simulink model "Simulazione_OSSERVATORE"  (R2022b)
settings: Solver=VariableStepAuto  StartTime=0.0  StopTime=20  RelTol=1e-10  AbsTol=1e-10
values from neighbouring files (symbols this model uses):
  A = [ 0    0     1     0 ... (first row only)    [Tirocinio3_main.m]
  A_d = A'    [ProgettoOsservatore.m]    (also in ProgettoOsservatoreOTTIMO.m; Tirocinio3_main.m = [ 0    0     1     0)
  B = [0 0 1/m1 0 ]'    [Tirocinio3_main.m]
  B_d = C'    [ProgettoOsservatoreOTTIMO.m]    (also in Tirocinio3_main.m = [0 0 1/m1_d 0 ]')
  C = [1 0 0 0]    [Tirocinio3_main.m]
  C_d = B'    [ProgettoOsservatore.m]    (also in Tirocinio3_main.m = [1 0 0 0])
  D = 0    [Tirocinio3_main.m]
  D_d = 0    [Tirocinio3_main.m]
  M = [0 0 0 1/m2]'    [Tirocinio3_main.m]
  V_ott = K'    [Tirocinio3_main.m]
  x0 = [x1; x2; v1 ; v2 ]    [Tirocinio3_main.m]
undefined symbols (not defined in the file or in its folder): V_fast, V_slow
libraries: simulink x2
settings Model: Creator=Danilo  LastModifiedBy=Danilo

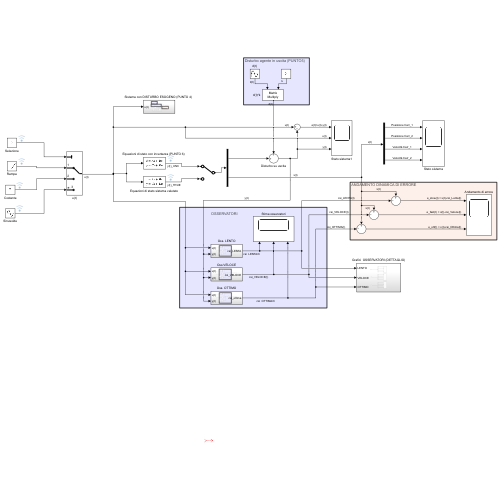
[thumbnail: Simulink's stored preview of the top-level diagram]
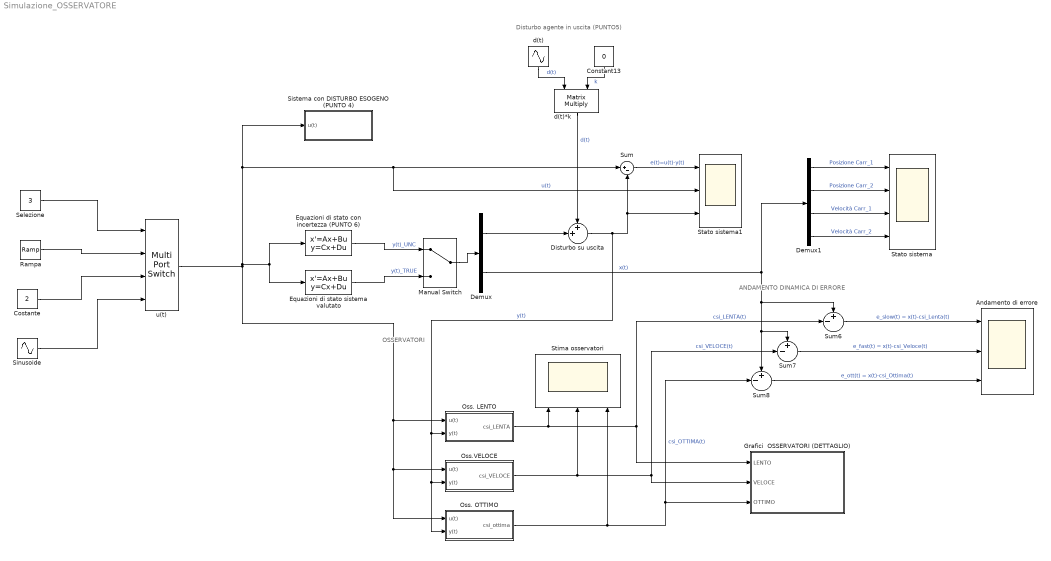
== system Simulazione_OSSERVATORE ==
  note: OSSERVATORI
  note: ANDAMENTO DINAMICA DI ERRORE
  note: Disturbo agente in uscita (PUNTO5)
  Andamento di errore : Scope  NumInputPorts=3
  Constant13 : Constant  Value=0  VectorParams1D=off
  Costante : Constant  Value=2
  Demux : Demux  Outputs=[1,4]
  Demux1 : Demux
  Disturbo su uscita : Sum  Inputs=++|
  "Equazioni di stato con incertezza (PUNTO 6)  " : StateSpace  A=A_d  B=B_d  C=[C_d ; eye(4)]  D=[D_d;zeros(4,1)]  InitialCondition=x0
  "Equazioni di stato sistema valutato " : StateSpace  A=A  B=B  C=[C ; eye(4)]  D=[D;zeros(4,1)]  InitialCondition=x0
  Grafici  OSSERVATORI (DETTAGLIO) : Subsystem
  Manual Switch : ManualSwitch
  Oss. LENTO : Subsystem
  Oss. OTTIMO : Subsystem
  Oss.VELOCE : Subsystem
  Rampa : simulink/Sources/Ramp  slope=5  start=0  InitialOutput=0
  Selezione : Constant  Value=3
  Sinusoide : Sin  SampleTime=0
  "Sistema con DISTURBO ESOGENO (PUNTO 4)  " : Subsystem
  Stato sistema : Scope  NumInputPorts=4
  Stato sistema1 : Scope  NumInputPorts=3
  Stima osservatori : Scope  NumInputPorts=3
  Sum : Sum  Inputs=|+-
  Sum6 : Sum  Inputs=+-|
  Sum7 : Sum  Inputs=+-|
  Sum8 : Sum  Inputs=+-|
  d(t) : Sin  Amplitude=0.5  Frequency=10  SampleTime=0
  d(t)*k : Product  Multiplication=Matrix(*)
  u(t) : MultiPortSwitch  SaturateOnIntegerOverflow=off  InputSameDT=off
  wires:
  Demux/1 -> Disturbo su uscita/2
  Oss. LENTO/1(csi_LENTA) -> Grafici  OSSERVATORI (DETTAGLIO)/1(LENTO), Sum6/2, Stima osservatori/1  "csi_LENTA(t)"
  Sinusoide/1 -> u(t)/4
  Rampa/1 -> u(t)/2
  Costante/1 -> u(t)/3
  Selezione/1 -> u(t)/1
  Sum/1 -> Stato sistema1/1  "e(t)=u(t)-y(t)"
  ? -> ?
  Oss. OTTIMO/1(csi_ottima) -> Sum8/2, Grafici  OSSERVATORI (DETTAGLIO)/3(OTTIMO), Stima osservatori/3  "csi_OTTIMA(t)"
  Sum8/1 -> Andamento di errore/3  "e_ott(t) = x(t)-csi_Ottima(t)"
  Sum6/1 -> Andamento di errore/1  "e_slow(t) = x(t)-csi_Lenta(t)"
  Sum7/1 -> Andamento di errore/2  "e_fast(t) = x(t)-csi_Veloce(t)"
  Demux/2 -> Sum6/1, Sum8/1, Sum7/1, Demux1/1  "x(t)"
  u(t)/1 -> Oss. OTTIMO/1(u(t)), Oss.VELOCE/1(u(t)), Oss. LENTO/1(u(t)), "Sistema con DISTURBO ESOGENO (PUNTO 4)  "/1(u(t)), Stato sistema1/2, Sum/1, "Equazioni di stato con incertezza (PUNTO 6)  "/1, "Equazioni di stato sistema valutato "/1  "u(t)"
  Oss.VELOCE/1(csi_VELOCE) -> Sum7/2, Grafici  OSSERVATORI (DETTAGLIO)/2(VELOCE), Stima osservatori/2  "csi_VELOCE(t)"
  Demux1/1 -> Stato sistema/1  "Posizione Carr_1"
  Demux1/4 -> Stato sistema/4  "Velocità Carr_2"
  Demux1/3 -> Stato sistema/3  "Velocità Carr_1"
  Demux1/2 -> Stato sistema/2  "Posizione Carr_2"
  d(t)/1 -> d(t)*k/1  "d(t)"
  Constant13/1 -> d(t)*k/2  "k"
  Disturbo su uscita/1 -> Sum/2, Stato sistema1/3, Oss. OTTIMO/2(y(t)), Oss.VELOCE/2(y(t)), Oss. LENTO/2(y(t))  "y(t)"
  d(t)*k/1 -> Disturbo su uscita/1  "d(t)"
  Manual Switch/1 -> Demux/1
  "Equazioni di stato sistema valutato "/1 -> Manual Switch/2  "y(t)_TRUE"
  "Equazioni di stato con incertezza (PUNTO 6)  "/1 -> Manual Switch/1  "y(t)_UNC"

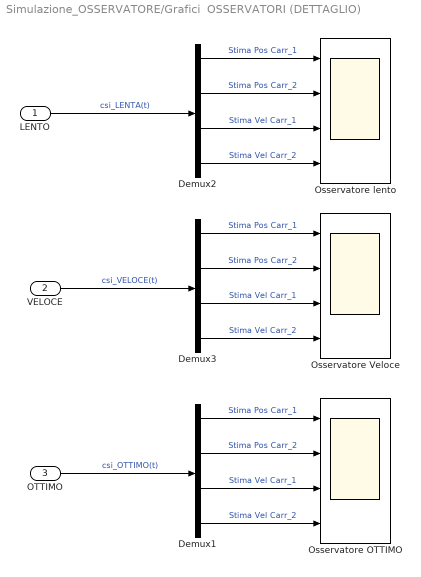
== system Simulazione_OSSERVATORE/Grafici  OSSERVATORI (DETTAGLIO) ==
  LENTO : Inport
  VELOCE : Inport  Port=2
  OTTIMO : Inport  Port=3
  Demux1 : Demux
  Demux2 : Demux
  Demux3 : Demux
  Osservatore OTTIMO : Scope  NumInputPorts=4
  Osservatore Veloce : Scope  NumInputPorts=4
  "Osservatore lento " : Scope  NumInputPorts=4
  wires:
  Demux1/3 -> Osservatore OTTIMO/3  "Stima Vel Carr_1"
  Demux1/4 -> Osservatore OTTIMO/4  "Stima Vel Carr_2"
  Demux1/2 -> Osservatore OTTIMO/2  "Stima Pos Carr_2"
  Demux3/4 -> Osservatore Veloce/4  "Stima Vel Carr_2"
  Demux3/2 -> Osservatore Veloce/2  "Stima Pos Carr_2"
  Demux3/3 -> Osservatore Veloce/3  "Stima Vel Carr_1"
  Demux3/1 -> Osservatore Veloce/1  "Stima Pos Carr_1"
  Demux1/1 -> Osservatore OTTIMO/1  "Stima Pos Carr_1"
  LENTO/1 -> Demux2/1  "csi_LENTA(t)"
  Demux2/2 -> "Osservatore lento "/2  "Stima Pos Carr_2"
  Demux2/4 -> "Osservatore lento "/4  "Stima Vel Carr_2"
  Demux2/3 -> "Osservatore lento "/3  "Stima Vel Carr_1"
  Demux2/1 -> "Osservatore lento "/1  "Stima Pos Carr_1"
  VELOCE/1 -> Demux3/1  "csi_VELOCE(t)"
  OTTIMO/1 -> Demux1/1  "csi_OTTIMO(t)"

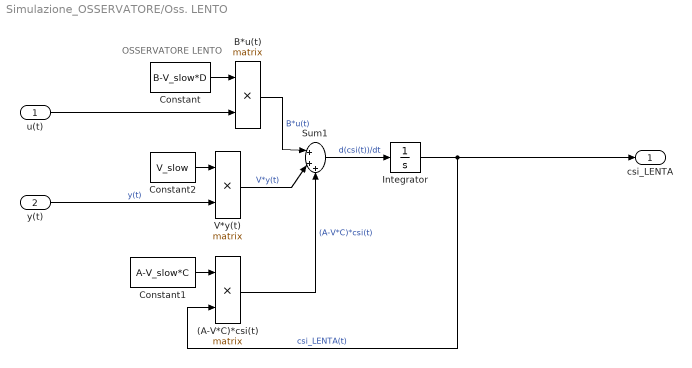
== system Simulazione_OSSERVATORE/Oss. LENTO ==
  note: OSSERVATORE LENTO
  u(t) : Inport
  y(t) : Inport  Port=2
  (A-V*C)*csi(t) : Product  Multiplication=Matrix(*)
  B*u(t) : Product  Multiplication=Matrix(*)
  Constant : Constant  Value=B-V_slow*D
  Constant1 : Constant  Value=A-V_slow*C
  Constant2 : Constant  Value=V_slow
  Integrator : Integrator  InitialCondition=x0
  Sum1 : Sum  Inputs=|+++
  V*y(t) : Product  Multiplication=Matrix(*)
  csi_LENTA : Outport
  wires:
  B*u(t)/1 -> Sum1/1  "B*u(t)"
  V*y(t)/1 -> Sum1/2  "V*y(t)"
  Constant/1 -> B*u(t)/1
  Sum1/1 -> Integrator/1  "d(csi(t))/dt"
  Constant2/1 -> V*y(t)/1
  y(t)/1 -> V*y(t)/2  "y(t)"
  Integrator/1 -> csi_LENTA/1, (A-V*C)*csi(t)/2  "csi_LENTA(t)"
  (A-V*C)*csi(t)/1 -> Sum1/3  "(A-V*C)*csi(t)"
  Constant1/1 -> (A-V*C)*csi(t)/1
  u(t)/1 -> B*u(t)/2

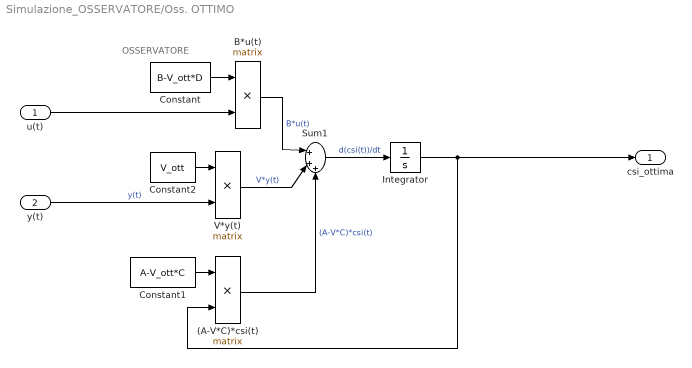
== system Simulazione_OSSERVATORE/Oss. OTTIMO ==
  note: OSSERVATORE
  u(t) : Inport
  y(t) : Inport  Port=2
  (A-V*C)*csi(t) : Product  Multiplication=Matrix(*)
  B*u(t) : Product  Multiplication=Matrix(*)
  Constant : Constant  Value=B-V_ott*D
  Constant1 : Constant  Value=A-V_ott*C
  Constant2 : Constant  Value=V_ott
  Integrator : Integrator  InitialCondition=x0
  Sum1 : Sum  Inputs=|+++
  V*y(t) : Product  Multiplication=Matrix(*)
  csi_ottima : Outport
  wires:
  B*u(t)/1 -> Sum1/1  "B*u(t)"
  V*y(t)/1 -> Sum1/2  "V*y(t)"
  Constant/1 -> B*u(t)/1
  Sum1/1 -> Integrator/1  "d(csi(t))/dt"
  Constant2/1 -> V*y(t)/1
  y(t)/1 -> V*y(t)/2  "y(t)"
  Integrator/1 -> csi_ottima/1, (A-V*C)*csi(t)/2
  (A-V*C)*csi(t)/1 -> Sum1/3  "(A-V*C)*csi(t)"
  Constant1/1 -> (A-V*C)*csi(t)/1
  u(t)/1 -> B*u(t)/2

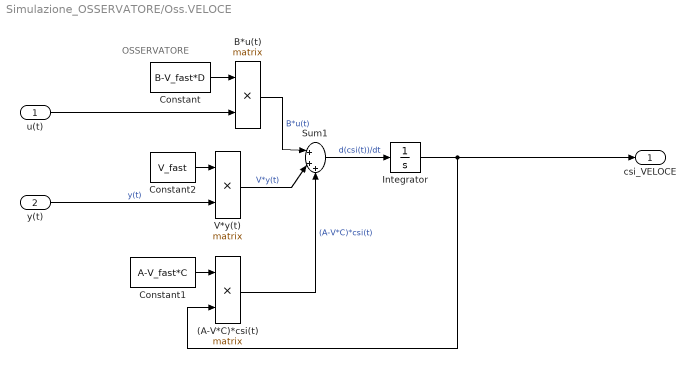
== system Simulazione_OSSERVATORE/Oss.VELOCE ==
  note: OSSERVATORE
  u(t) : Inport
  y(t) : Inport  Port=2
  (A-V*C)*csi(t) : Product  Multiplication=Matrix(*)
  B*u(t) : Product  Multiplication=Matrix(*)
  Constant : Constant  Value=B-V_fast*D
  Constant1 : Constant  Value=A-V_fast*C
  Constant2 : Constant  Value=V_fast
  Integrator : Integrator  InitialCondition=x0
  Sum1 : Sum  Inputs=|+++
  V*y(t) : Product  Multiplication=Matrix(*)
  csi_VELOCE : Outport
  wires:
  B*u(t)/1 -> Sum1/1  "B*u(t)"
  V*y(t)/1 -> Sum1/2  "V*y(t)"
  Constant/1 -> B*u(t)/1
  Sum1/1 -> Integrator/1  "d(csi(t))/dt"
  Constant2/1 -> V*y(t)/1
  y(t)/1 -> V*y(t)/2  "y(t)"
  Integrator/1 -> csi_VELOCE/1, (A-V*C)*csi(t)/2
  (A-V*C)*csi(t)/1 -> Sum1/3  "(A-V*C)*csi(t)"
  Constant1/1 -> (A-V*C)*csi(t)/1
  u(t)/1 -> B*u(t)/2

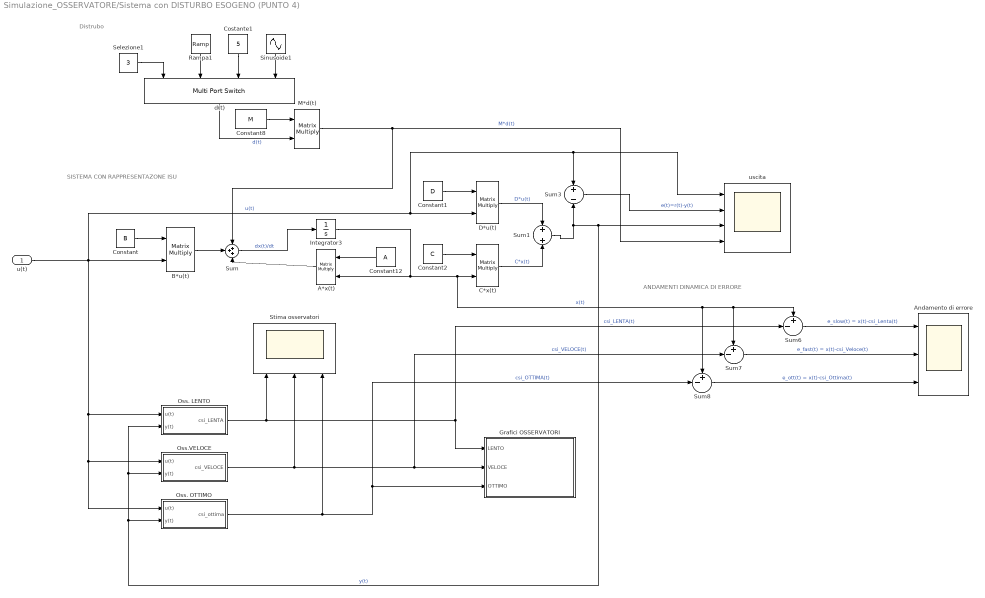
== system Simulazione_OSSERVATORE/Sistema con DISTURBO ESOGENO (PUNTO 4)   ==
  note: ANDAMENTI DINAMICA DI ERRORE
  note: Distrubo
  note: SISTEMA CON RAPPRESENTAZONE ISU
  u(t) : Inport
  A*x(t) : Product  Multiplication=Matrix(*)
  Andamento di errore : Scope  NumInputPorts=3
  B*u(t) : Product  Multiplication=Matrix(*)
  C*x(t) : Product  Multiplication=Matrix(*)
  Constant : Constant  Value=B  VectorParams1D=off
  Constant1 : Constant  Value=D  VectorParams1D=off
  Constant12 : Constant  Value=A  VectorParams1D=off
  Constant2 : Constant  Value=C  VectorParams1D=off
  Constant8 : Constant  Value=M
  Costante1 : Constant  Value=5
  D*u(t) : Product  Multiplication=Matrix(*)
  Grafici OSSERVATORI : Subsystem
  Integrator3 : Integrator
  M*d(t) : Product  Multiplication=Matrix(*)
  Oss. LENTO : Subsystem
  Oss. OTTIMO : Subsystem
  Oss.VELOCE : Subsystem
  Rampa1 : simulink/Sources/Ramp  slope=5  start=0  InitialOutput=0
  Selezione1 : Constant  Value=3
  Sinusoide1 : Sin  Amplitude=5  Frequency=5  SampleTime=0
  Stima osservatori : Scope  NumInputPorts=3
  Sum : Sum  Inputs=+++
  Sum1 : Sum
  Sum3 : Sum  Inputs=+-
  Sum6 : Sum  Inputs=+-|
  Sum7 : Sum  Inputs=+-|
  Sum8 : Sum  Inputs=+-|
  d(t) : MultiPortSwitch  SaturateOnIntegerOverflow=off  InputSameDT=off
  uscita : Scope  NumInputPorts=4
  wires:
  Sum7/1 -> Andamento di errore/2  "e_fast(t) = x(t)-csi_Veloce(t)"
  Sum6/1 -> Andamento di errore/1  "e_slow(t) = x(t)-csi_Lenta(t)"
  Selezione1/1 -> d(t)/1
  Constant1/1 -> D*u(t)/1
  Sum/1 -> Integrator3/1  "dx(t)/dt"
  B*u(t)/1 -> Sum/2
  C*x(t)/1 -> Sum1/2  "C*x(t)"
  Sum3/1 -> uscita/2  "e(t)=r(t)-y(t)"
  Sum8/1 -> Andamento di errore/3  "e_ott(t) = x(t)-csi_Ottima(t)"
  Constant2/1 -> C*x(t)/1
  Integrator3/1 -> C*x(t)/2, Sum6/1, Sum7/1, Sum8/1, A*x(t)/2  "x(t)"
  M*d(t)/1 -> uscita/4, Sum/1  "M*d(t)"
  Sinusoide1/1 -> d(t)/4
  Rampa1/1 -> d(t)/2
  d(t)/1 -> M*d(t)/2  "d(t)"
  A*x(t)/1 -> Sum/3
  Costante1/1 -> d(t)/3
  Sum1/1 -> Sum3/2, Oss. OTTIMO/2(y(t)), Oss.VELOCE/2(y(t)), Oss. LENTO/2(y(t)), uscita/3  "y(t)"
  Constant8/1 -> M*d(t)/1
  D*u(t)/1 -> Sum1/1  "D*u(t)"
  Constant/1 -> B*u(t)/1
  Constant12/1 -> A*x(t)/1
  Oss.VELOCE/1(csi_VELOCE) -> Sum7/2, Grafici OSSERVATORI/2(VELOCE), Stima osservatori/2  "csi_VELOCE(t)"
  Oss. OTTIMO/1(csi_ottima) -> Sum8/2, Grafici OSSERVATORI/3(OTTIMO), Stima osservatori/3  "csi_OTTIMA(t)"
  Oss. LENTO/1(csi_LENTA) -> Sum6/2, Grafici OSSERVATORI/1(LENTO), Stima osservatori/1  "csi_LENTA(t)"
  u(t)/1 -> Oss. LENTO/1(u(t)), Oss.VELOCE/1(u(t)), Oss. OTTIMO/1(u(t)), Sum3/1, uscita/1, D*u(t)/2, B*u(t)/2  "u(t)"

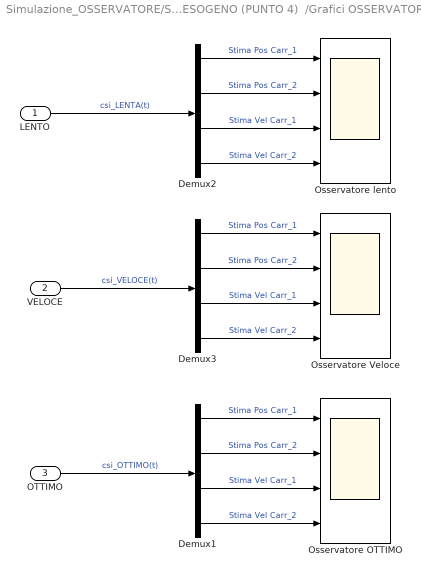
== system Simulazione_OSSERVATORE/Sistema con DISTURBO ESOGENO (PUNTO 4)  /Grafici OSSERVATORI ==
  LENTO : Inport
  VELOCE : Inport  Port=2
  OTTIMO : Inport  Port=3
  Demux1 : Demux
  Demux2 : Demux
  Demux3 : Demux
  Osservatore OTTIMO : Scope  NumInputPorts=4
  Osservatore Veloce : Scope  NumInputPorts=4
  "Osservatore lento " : Scope  NumInputPorts=4
  wires:
  Demux1/3 -> Osservatore OTTIMO/3  "Stima Vel Carr_1"
  Demux1/4 -> Osservatore OTTIMO/4  "Stima Vel Carr_2"
  Demux1/2 -> Osservatore OTTIMO/2  "Stima Pos Carr_2"
  Demux3/4 -> Osservatore Veloce/4  "Stima Vel Carr_2"
  Demux3/2 -> Osservatore Veloce/2  "Stima Pos Carr_2"
  Demux3/3 -> Osservatore Veloce/3  "Stima Vel Carr_1"
  Demux3/1 -> Osservatore Veloce/1  "Stima Pos Carr_1"
  Demux1/1 -> Osservatore OTTIMO/1  "Stima Pos Carr_1"
  LENTO/1 -> Demux2/1  "csi_LENTA(t)"
  Demux2/2 -> "Osservatore lento "/2  "Stima Pos Carr_2"
  Demux2/4 -> "Osservatore lento "/4  "Stima Vel Carr_2"
  Demux2/3 -> "Osservatore lento "/3  "Stima Vel Carr_1"
  Demux2/1 -> "Osservatore lento "/1  "Stima Pos Carr_1"
  VELOCE/1 -> Demux3/1  "csi_VELOCE(t)"
  OTTIMO/1 -> Demux1/1  "csi_OTTIMO(t)"

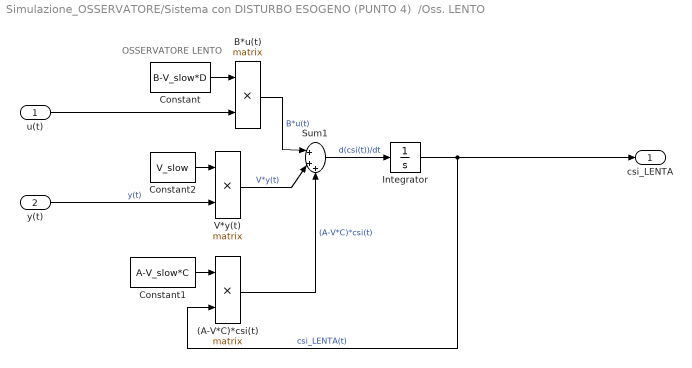
== system Simulazione_OSSERVATORE/Sistema con DISTURBO ESOGENO (PUNTO 4)  /Oss. LENTO ==
  note: OSSERVATORE LENTO
  u(t) : Inport
  y(t) : Inport  Port=2
  (A-V*C)*csi(t) : Product  Multiplication=Matrix(*)
  B*u(t) : Product  Multiplication=Matrix(*)
  Constant : Constant  Value=B-V_slow*D
  Constant1 : Constant  Value=A-V_slow*C
  Constant2 : Constant  Value=V_slow
  Integrator : Integrator  InitialCondition=x0
  Sum1 : Sum  Inputs=|+++
  V*y(t) : Product  Multiplication=Matrix(*)
  csi_LENTA : Outport
  wires:
  B*u(t)/1 -> Sum1/1  "B*u(t)"
  V*y(t)/1 -> Sum1/2  "V*y(t)"
  Constant/1 -> B*u(t)/1
  Sum1/1 -> Integrator/1  "d(csi(t))/dt"
  Constant2/1 -> V*y(t)/1
  y(t)/1 -> V*y(t)/2  "y(t)"
  Integrator/1 -> csi_LENTA/1, (A-V*C)*csi(t)/2  "csi_LENTA(t)"
  (A-V*C)*csi(t)/1 -> Sum1/3  "(A-V*C)*csi(t)"
  Constant1/1 -> (A-V*C)*csi(t)/1
  u(t)/1 -> B*u(t)/2

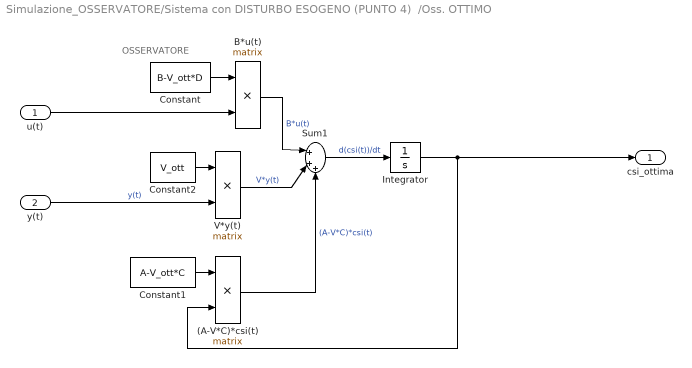
== system Simulazione_OSSERVATORE/Sistema con DISTURBO ESOGENO (PUNTO 4)  /Oss. OTTIMO ==
  note: OSSERVATORE
  u(t) : Inport
  y(t) : Inport  Port=2
  (A-V*C)*csi(t) : Product  Multiplication=Matrix(*)
  B*u(t) : Product  Multiplication=Matrix(*)
  Constant : Constant  Value=B-V_ott*D
  Constant1 : Constant  Value=A-V_ott*C
  Constant2 : Constant  Value=V_ott
  Integrator : Integrator  InitialCondition=x0
  Sum1 : Sum  Inputs=|+++
  V*y(t) : Product  Multiplication=Matrix(*)
  csi_ottima : Outport
  wires:
  B*u(t)/1 -> Sum1/1  "B*u(t)"
  V*y(t)/1 -> Sum1/2  "V*y(t)"
  Constant/1 -> B*u(t)/1
  Sum1/1 -> Integrator/1  "d(csi(t))/dt"
  Constant2/1 -> V*y(t)/1
  y(t)/1 -> V*y(t)/2  "y(t)"
  Integrator/1 -> csi_ottima/1, (A-V*C)*csi(t)/2
  (A-V*C)*csi(t)/1 -> Sum1/3  "(A-V*C)*csi(t)"
  Constant1/1 -> (A-V*C)*csi(t)/1
  u(t)/1 -> B*u(t)/2

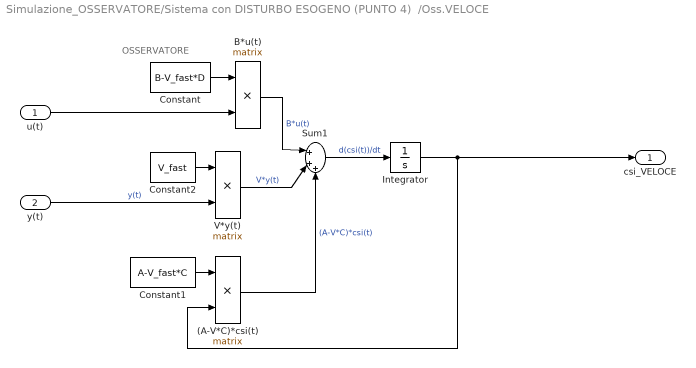
== system Simulazione_OSSERVATORE/Sistema con DISTURBO ESOGENO (PUNTO 4)  /Oss.VELOCE ==
  note: OSSERVATORE
  u(t) : Inport
  y(t) : Inport  Port=2
  (A-V*C)*csi(t) : Product  Multiplication=Matrix(*)
  B*u(t) : Product  Multiplication=Matrix(*)
  Constant : Constant  Value=B-V_fast*D
  Constant1 : Constant  Value=A-V_fast*C
  Constant2 : Constant  Value=V_fast
  Integrator : Integrator  InitialCondition=x0
  Sum1 : Sum  Inputs=|+++
  V*y(t) : Product  Multiplication=Matrix(*)
  csi_VELOCE : Outport
  wires:
  B*u(t)/1 -> Sum1/1  "B*u(t)"
  V*y(t)/1 -> Sum1/2  "V*y(t)"
  Constant/1 -> B*u(t)/1
  Sum1/1 -> Integrator/1  "d(csi(t))/dt"
  Constant2/1 -> V*y(t)/1
  y(t)/1 -> V*y(t)/2  "y(t)"
  Integrator/1 -> csi_VELOCE/1, (A-V*C)*csi(t)/2
  (A-V*C)*csi(t)/1 -> Sum1/3  "(A-V*C)*csi(t)"
  Constant1/1 -> (A-V*C)*csi(t)/1
  u(t)/1 -> B*u(t)/2
